simulink model "controller"  (R2021b)
settings: Solver=FixedStepDiscrete  StartTime=0.0  StopTime=10.0  FixedStep=0.001  RelTol=1e-3  EnableMultiTasking=on
undefined symbols (not defined in the file): DiscIntNeverNeededParam
settings Model: Creator=david  LastModifiedBy=david

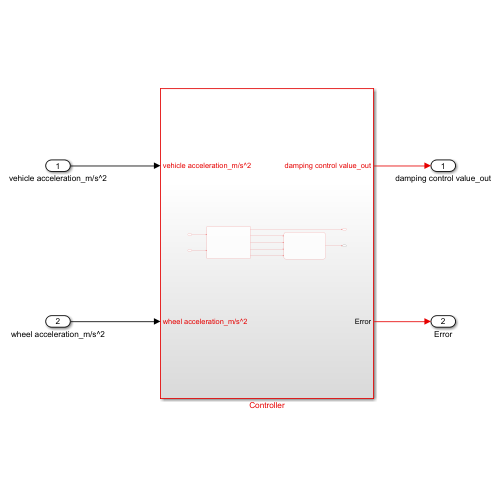
[thumbnail: Simulink's stored preview of the top-level diagram]
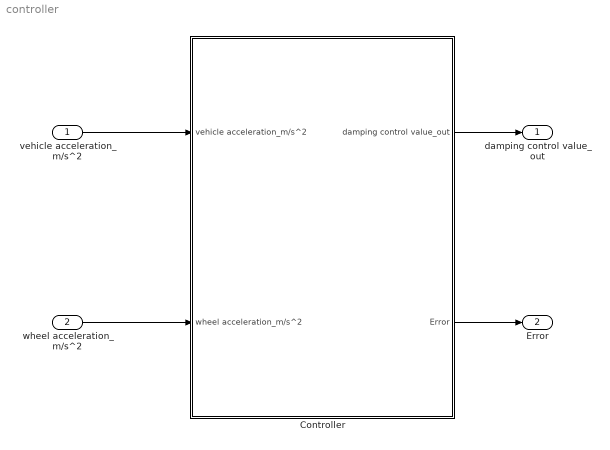
== system controller ==
  vehicle acceleration_m/s^2 : Inport
  wheel acceleration_m/s^2 : Inport  Port=2
  Controller : Subsystem
  damping control value_out : Outport  VectorParamsAs1DForOutWhenUnconnected=on
  Error : Outport  Port=2  VectorParamsAs1DForOutWhenUnconnected=on
  wires:
  vehicle acceleration_m/s^2/1 -> Controller/1(vehicle acceleration_m/s^2)
  wheel acceleration_m/s^2/1 -> Controller/2(wheel acceleration_m/s^2)
  Controller/1(damping control value_out) -> damping control value_out/1
  Controller/2(Error) -> Error/1

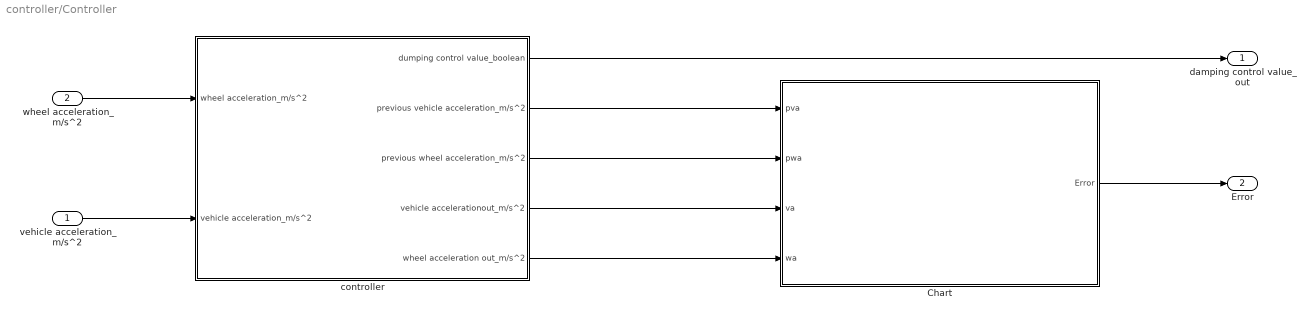
== system controller/Controller ==
  vehicle acceleration_m/s^2 : Inport  OutDataTypeStr=double  Unit=m/s^2  PortDimensions=1
  wheel acceleration_m/s^2 : Inport  Port=2  OutDataTypeStr=double  Unit=m/s^2  PortDimensions=1
  Chart : Stateflow chart  TreatAsAtomicUnit=on
  controller : Subsystem
  damping control value_out : Outport  OutDataTypeStr=uint8  PortDimensions=1
  Error : Outport  Port=2  VectorParamsAs1DForOutWhenUnconnected=on
  wires:
  vehicle acceleration_m/s^2/1 -> controller/2(vehicle acceleration_m/s^2)
  wheel acceleration_m/s^2/1 -> controller/1(wheel acceleration_m/s^2)
  Chart/1(Error) -> Error/1
  controller/1(dumping control value_boolean) -> damping control value_out/1
  controller/2(previous vehicle acceleration_m/s^2) -> Chart/1(pva)
  controller/3(previous wheel acceleration_m/s^2) -> Chart/2(pwa)
  controller/4(vehicle accelerationout_m/s^2) -> Chart/3(va)
  controller/5(wheel acceleration out_m/s^2) -> Chart/4(wa)

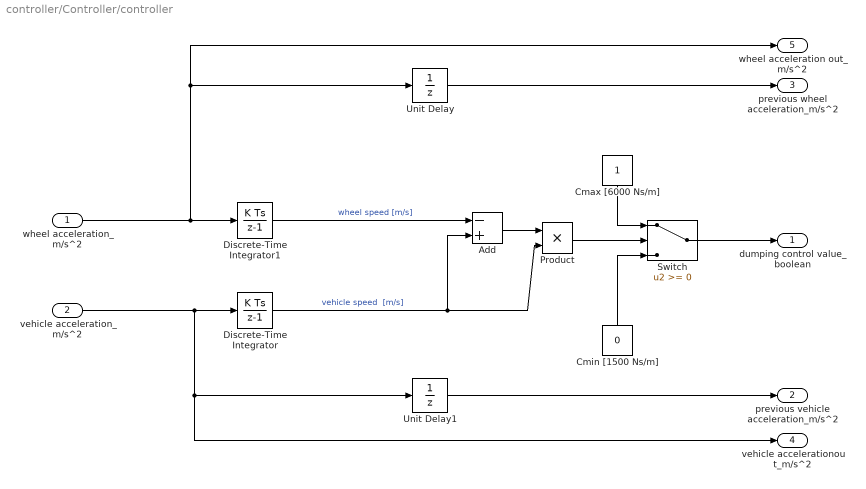
== system controller/Controller/controller ==
  wheel acceleration_m/s^2 : Inport
  vehicle acceleration_m/s^2 : Inport  Port=2  OutDataTypeStr=double  PortDimensions=1
  Add : Sum  Inputs=-+
  Cmax [6000 Ns/m] : Constant  OutDataTypeStr=uint8
  Cmin [1500 Ns/m] : Constant  Value=0  OutDataTypeStr=uint8
  Discrete-Time Integrator : DiscreteIntegrator  SampleTime=-1  ICPrevOutput=DiscIntNeverNeededParam  ICPrevScaledInput=DiscIntNeverNeededParam
  Discrete-Time Integrator1 : DiscreteIntegrator  SampleTime=-1  ICPrevOutput=DiscIntNeverNeededParam  ICPrevScaledInput=DiscIntNeverNeededParam
  Product : Product
  Switch : Switch
  Unit Delay : UnitDelay  SampleTime=-1  HasFrameUpgradeWarning=on
  Unit Delay1 : UnitDelay  SampleTime=-1  HasFrameUpgradeWarning=on
  dumping control value_boolean : Outport  OutDataTypeStr=uint8
  previous vehicle acceleration_m/s^2 : Outport  Port=2  VectorParamsAs1DForOutWhenUnconnected=on
  previous wheel acceleration_m/s^2 : Outport  Port=3  VectorParamsAs1DForOutWhenUnconnected=on
  vehicle accelerationout_m/s^2 : Outport  Port=4  VectorParamsAs1DForOutWhenUnconnected=on
  wheel acceleration out_m/s^2 : Outport  Port=5  VectorParamsAs1DForOutWhenUnconnected=on
  wires:
  wheel acceleration_m/s^2/1 -> wheel acceleration out_m/s^2/1, Unit Delay/1, Discrete-Time Integrator1/1
  Cmax [6000 Ns/m]/1 -> Switch/1
  Cmin [1500 Ns/m]/1 -> Switch/3
  Discrete-Time Integrator/1 -> Product/2, Add/2  "vehicle speed  [m/s]"
  Add/1 -> Product/1
  vehicle acceleration_m/s^2/1 -> vehicle accelerationout_m/s^2/1, Unit Delay1/1, Discrete-Time Integrator/1
  Product/1 -> Switch/2
  Discrete-Time Integrator1/1 -> Add/1  "wheel speed [m/s]"
  Unit Delay/1 -> previous wheel acceleration_m/s^2/1
  Unit Delay1/1 -> previous vehicle acceleration_m/s^2/1
  Switch/1 -> dumping control value_boolean/1

== stateflow chart controller/Controller/Chart ==
  state ErrorLogic
    state NO_ERROR
      en:
      Error=0;
    state CHECK_STATE
    state ERROR
      en:
      Error=1
    (default) -> NO_ERROR
    NO_ERROR -> CHECK_STATE
    CHECK_STATE -> ERROR [order 1] : after(20,msec)
    CHECK_STATE -> NO_ERROR [order 2] : [(va) ~= (pva) && (wa) ~= (pwa)]
  data: pva input double; pwa input double; va input double; wa input double; Error output uint8
